simulink model "pulchan_r2"  (R2012b)
(part 2 of 91)

  sampling_frequency_mhz/1(sim_reg_out) -> Terminator24/1
  Constant17/1 -> Delay34/1
  Delay34/1 -> sampling_frequency_mhz/1(reg_out)
  coarse_fft_size_nsamp/1(sim_reg_out) -> Terminator25/1
  Constant18/1 -> Delay35/1
  Delay35/1 -> coarse_fft_size_nsamp/1(reg_out)
  fine_fft_size_nsamp/1(sim_reg_out) -> Terminator26/1
  Constant19/1 -> Delay36/1
  Delay36/1 -> fine_fft_size_nsamp/1(reg_out)
  Constant1/1 -> adc0_en/1(sim_1)
  Constant4/1 -> adc0_atten/1(sim_1)
  Constant2/1 -> adc1_en/1(sim_1)
  Constant3/1 -> adc1_atten/1(sim_1)
  noise_diode_en/1(in_reg) -> Terminator28/1
  Constant28/1 -> noise_diode_en/1(sim_1)
  noise_diode_duty_cycle_en/1(in_reg) -> Terminator29/1
  Constant29/1 -> noise_diode_duty_cycle_en/1(sim_1)
  noise_diode_on_length/1(in_reg) -> Terminator30/1
  Constant30/1 -> noise_diode_on_length/1(sim_1)
  noise_diode_off_length/1(in_reg) -> Terminator38/1
  Constant32/1 -> noise_diode_off_length/1(sim_1)
  Delay30/1 -> tengbe0/6(tx_end_of_frame)
  Delay33/1 -> tengbe1/6(tx_end_of_frame)
  Gateway Out1/1 -> Scope/1  "sync_in"
  Gateway Out/1 -> Scope/2  "dv_in"
  Gateway Out2/1 -> Scope/3  "dv_out"
  [use_self_pps] -> Delay39/1
